simulink model "fromWorkSpace_TestGen3"  (R2017b)
settings: Solver=FixedStepDiscrete  StartTime=0.0  StopTime=10.0  RelTol=1e-3
model workspace (MAT data in the model file):
  X_matrix = [0 0.2 0.4 0.6 0.8 1 1.2 1.4 1.6 1.8 2 2.2 ... (200 elements, 50x4)]
undefined symbols (not defined in the file): Block_TestLib, reset
settings Model: Creator=ktrinh  LastModifiedBy=ktrinh
settings DebuggingCC: ParameterOverflowMsg=none

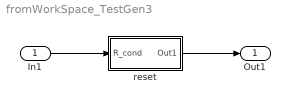
== system fromWorkSpace_TestGen3 ==
  In1 : Inport
  reset : Subsystem  AncestorBlock=Block_TestLib/reset
  Out1 : Outport
  wires:
  In1/1 -> reset/1(R_cond)
  reset/1(Out1) -> Out1/1

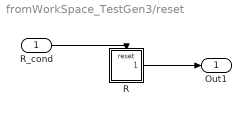
== system fromWorkSpace_TestGen3/reset ==
  R_cond : Inport  OutDataTypeStr=boolean
  R : Subsystem  TreatAsAtomicUnit=on
  Out1 : Outport
  wires:
  R_cond/1 -> R/Reset
  R/1(Out1) -> Out1/1

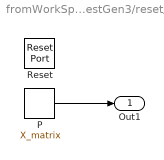
== system fromWorkSpace_TestGen3/reset/R ==
  Reset : ResetPort  DisableCoverage=on
  P : FromWorkspace  VariableName=X_matrix  Interpolate=off  OutputAfterFinalValue=Holding final value
  Out1 : Outport
  wires:
  P/1 -> Out1/1
